simulink model "roll_ap"  (R2017b)
settings: Solver=FixedStepDiscrete  StartTime=0.0  StopTime=25  FixedStep=1/40  RelTol=1e-3
model workspace (MAT data in the model file):
  dispGain = Simulink.Parameter
  dispGain.Value = 1
  dispGain.DataType = 'auto'
  dispGain.Dimensions = [1 1]
  hdgGain = Simulink.Parameter
  hdgGain.Value = 0.015
  hdgGain.DataType = 'auto'
  hdgGain.Min = 0
  hdgGain.Dimensions = [1 1]
  intGain = Simulink.Parameter
  intGain.Value = 1
  intGain.DataType = 'auto'
  intGain.Dimensions = [1 1]
  rateGain = Simulink.Parameter
  rateGain.Value = 3
  rateGain.DataType = 'auto'
  rateGain.Dimensions = [1 1]
undefined symbols (not defined in the file or in its folder): cmdLim, dispLim, intLim, rateLim
libraries: simulink x1, simulink_need_slupdate x1
settings Model: RequirementInfo={} %GIDa_fe9045fd_0412_4b6e_8206_617cc20e6fde  ParameterArgumentNames=dispGain,intGain,rateGain,hdgGain  Creator=bpotter  LastModifiedBy=Hualong Yu
settings DataIOCC: ExternalInput=rollIn  SaveFormat=StructureWithTime  SignalLoggingSaveFormat=ModelDataLogs  SaveOutput=off  SignalLogging=off  SaveTime=off  OutputSaveName=Ail_Cmd
settings OptimizationCC: BlockReduction=off  DefaultParameterBehavior=Inlined  InlineInvariantSignals=on  ExpressionDepthLimit=2147483647  EfficientFloat2IntCast=on  EfficientMapNaN2IntZero=off  LifeSpan=inf  MaxStackSize=inf
settings DebuggingCC: SignalInfNanChecking=error  SignalRangeChecking=error  ReadBeforeWriteMsg=EnableAllAsError  WriteAfterWriteMsg=EnableAllAsError  WriteAfterReadMsg=EnableAllAsError  AlgebraicLoopMsg=error  ArtificialAlgebraicLoopMsg=error  SaveWithDisabledLinksMsg=error  SaveWithParameterizedLinksMsg=error  CheckExecutionContextPreStartOutputMsg=on  CheckExecutionContextRuntimeOutputMsg=on  BlockPriorityViolationMsg=error  MaxConsecutiveZCsMsg=warning  SolverPrmCheckMsg=error  InheritedTsInSrcMsg=error  SingleTaskRateTransMsg=error  TasksWithSamePriorityMsg=error  SigSpecEnsureSampleTimeMsg=error  CheckMatrixSingularityMsg=error  IntegerOverflowMsg=error  ParameterUnderflowMsg=error  ParameterPrecisionLossMsg=error  ParameterTunabilityLossMsg=error  UnderSpecifiedDataTypeMsg=error  UnnecessaryDatatypeConvMsg=warning  VectorMatrixConversionMsg=error  SignalLabelMismatchMsg=error  UnconnectedInputMsg=error  UnconnectedOutputMsg=error  UnconnectedLineMsg=error  SFcnCompatibilityMsg=error  UniqueDataStoreMsg=error  BusObjectLabelMismatch=error  RootOutportRequireBusObject=error  AssertControl=DisableAll  ModelReferenceIOMsg=error  ModelReferenceIOMismatchMessage=error  UnknownTsInhSupMsg=error  ModelReferenceDataLoggingMessage=error  ModelReferenceExtraNoncontSigs=none  StateNameClashWarn=warning  StrictBusMsg=ErrorOnBusTreatedAsVector  NonBusSignalsTreatedAsBus=error  SFUnexpectedBacktrackingDiag=warning  SFNoUnconditionalDefaultTransitionDiag=warning  SFExecutionAtInitializationDiag=none  IntegerSaturationMsg=error
settings HardwareCC: ProdBitPerPointer=32  ProdBitPerSizeT=32  ProdBitPerPtrDiffT=32  ProdLargestAtomicFloat=None  ProdEndianess=BigEndian  ProdWordSize=32  ProdHWDeviceType=32-bit Embedded Processor  TargetHWDeviceType=32-bit Generic
settings ModelReferenceCC: PropagateSignalLabelsOutOfModel=off
settings SFSimCC: MATLABDynamicMemAlloc=off
settings RTWCC: SystemTargetFile=ert.tlc  GenCodeOnly=on  GenerateMakefile=off  TemplateMakefile=ert_default_tmf  GenerateReport=on  RTWVerbose=off  IncludeHyperlinkInReport=on  LaunchReport=on  GenerateTraceInfo=on  GenerateTraceReport=on  GenerateTraceReportSl=on  GenerateTraceReportSf=on  GenerateTraceReportEml=on
settings CodeAppCC: ForceParamTrailComments=on  IgnoreCustomStorageClasses=off  MaxIdLength=63  MangleLength=4  CustomSymbolStrType=$N$R$M  StateflowObjectComments=on  InternalIdentifier=Classic  ReqsInCode=on
settings ERTTargetCC: UtilityFuncGeneration=Shared location  MultiwordLength=2048  IncludeMdlTerminateFcn=off  GeneratePreprocessorConditionals=Disable all  SuppressErrorStatus=on  SupportAbsoluteTime=off  MultiInstanceERTCode=on  CodeInterfacePackaging=Reusable function  SupportNonFinite=off  SupportComplex=off  ParenthesesLevel=Maximum  MultiInstanceErrorCode=None  ERTCustomFileTemplate=example_file_process.tlc  PreserveExpressionOrder=on  PreserveIfCondition=on  ConvertIfToSwitch=off  SuppressUnreachableDefaultCases=off
settings ConfigComp: CovSaveName=covdata_rollAP  CovMetricSettings=dcmtrwe  CovHTMLOptions=-aTS=1 -bRG=1 -bTC=1 -hTR=1 -nFC=0 -scm=1 -bcm=1  CovSaveCumulativeToWorkspaceVar=on  CovSaveSingleToWorkspaceVar=on  CovCumulativeVarName=covCumulativeData_rollAP  CovCumulativeReport=on  CovReportOnPause=off  CovExternalEMLEnable=off

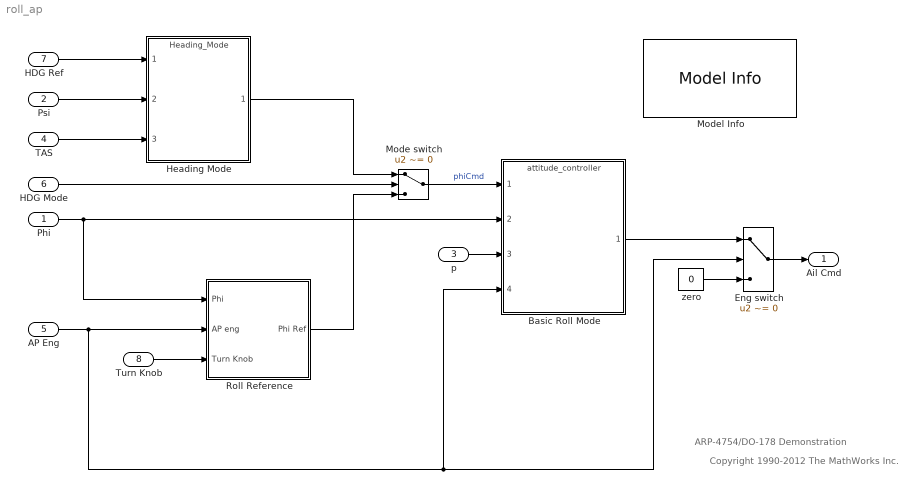
== system roll_ap ==
  note: Copyright 1990-2012 The MathWorks Inc.
  note: ARP-4754/DO-178 Demonstration
  Phi : Inport  RequirementInfo={} %GIDa_040c2d73_6311_42f9_964f_56f1fff3d8d8  OutDataTypeStr=double  PortDimensions=1  SampleTime=1/40  Interpolate=off
  Psi : Inport  RequirementInfo={} %GIDa_aa699f91_96f0_401b_acdb_f9b4b0743533  Port=2  OutDataTypeStr=double  PortDimensions=1  SampleTime=1/40  Interpolate=off
  p : Inport  RequirementInfo={} %GIDa_91b6e343_cedd_4c09_9e82_9cc09e4312a7  Port=3  OutDataTypeStr=double  PortDimensions=1  SampleTime=1/40  Interpolate=off
  TAS : Inport  RequirementInfo={} %GIDa_9daa2c3d_09c1_4ac6_a206_1425f5f778cd  Port=4  OutDataTypeStr=double  PortDimensions=1  SampleTime=1/40  Interpolate=off
  AP Eng : Inport  RequirementInfo={} %GIDa_dbf8c750_871c_42fc_8ea1_57838e97fa97  Port=5  OutDataTypeStr=boolean  PortDimensions=1  SampleTime=1/40  Interpolate=off
  HDG Mode : Inport  RequirementInfo={} %GIDa_3d1fd2be_b046_42ef_8f3c_1955bceadbb7  Port=6  OutDataTypeStr=boolean  PortDimensions=1  SampleTime=1/40  Interpolate=off
  HDG Ref : Inport  RequirementInfo={} %GIDa_96162cda_cb1a_490e_8dac_f861526aad50  Port=7  OutDataTypeStr=double  PortDimensions=1  SampleTime=1/40  Interpolate=off
  Turn Knob : Inport  RequirementInfo={} %GIDa_fa976ccd_1ea9_4823_b673_fef2768ad601  Port=8  OutDataTypeStr=double  PortDimensions=1  SampleTime=1/40  Interpolate=off
  Basic Roll Mode : ModelReference  RequirementInfo={} %GIDa_94fed7b0_f432_43f5_a2d9_2abccf075f5b  ModelNameDialog=attitude_controller  ParameterArgumentNames=cmdLim,dispGain,dispLim,intGain,intLim,rateGain,rateLim  ParameterArgumentValues=15,dispGain,30,intGain,5,rateGain,6  UsingDefaultArgumentValue=0,0,0,0,0,0,0  SimulationMode=Normal  ModelReferenceVersion=1.44
  Eng switch : Switch  RequirementInfo={} %GIDa_1f89e2a1_f10b_411b_80f1_4c7070559f04  Criteria=u2 ~= 0
  Heading Mode : ModelReference  RequirementInfo={} %GIDa_e0954c89_e814_46d2_8f67_6d4b1cdfab81  ModelNameDialog=Heading_Mode  ParameterArgumentNames=hdgGain  ParameterArgumentValues=hdgGain  UsingDefaultArgumentValue=0  SimulationMode=Normal  ModelReferenceVersion=1.133
  Mode switch : Switch  RequirementInfo={} %GIDa_89518de0_411a_4ee8_869d_c7ed5e5087e3  Criteria=u2 ~= 0
  Model Info : simulink/Model-Wide Utilities/Model Info  RequirementInfo={} %GIDa_ca11a4b2_f22f_461f_8532_eb2c7aa53101  Frame=on  DisplayStringWithTags=|  HorizontalTextAlignment=Left  LeftAlignmentValue=0.02
      | Roll Autopilot
      | Author: %<LastModifiedBy>
      | Model Version: %<ModelVersion>
      | Date: %<LastModificationDate>
  Roll Reference : Subsystem  TreatAsAtomicUnit=on
      settings: RTWSystemCode=Inline
  zero : Constant  RequirementInfo={} %GIDa_8c99e557_6257_4659_beae_770a67a6ac3a  Value=0  OutDataTypeStr=double
  Ail Cmd : Outport  RequirementInfo={} %GIDa_02b61f6d_71d4_4b0d_89ac_bfbca808eb5f  OutDataTypeStr=double  PortDimensions=1  SampleTime=1/40
  wires:
  HDG Ref/1 -> Heading Mode/1
  Phi/1 -> Roll Reference/1(Phi), Basic Roll Mode/2
  p/1 -> Basic Roll Mode/3
  Psi/1 -> Heading Mode/2
  TAS/1 -> Heading Mode/3
  Mode switch/1 -> Basic Roll Mode/1  "phiCmd"
  HDG Mode/1 -> Mode switch/2
  Heading Mode/1 -> Mode switch/1
  AP Eng/1 -> Eng switch/2, Basic Roll Mode/4, Roll Reference/2(AP eng)
  Basic Roll Mode/1 -> Eng switch/1
  Eng switch/1 -> Ail Cmd/1
  zero/1 -> Eng switch/3
  Roll Reference/1(Phi Ref) -> Mode switch/3
  Turn Knob/1 -> Roll Reference/3(Turn Knob)

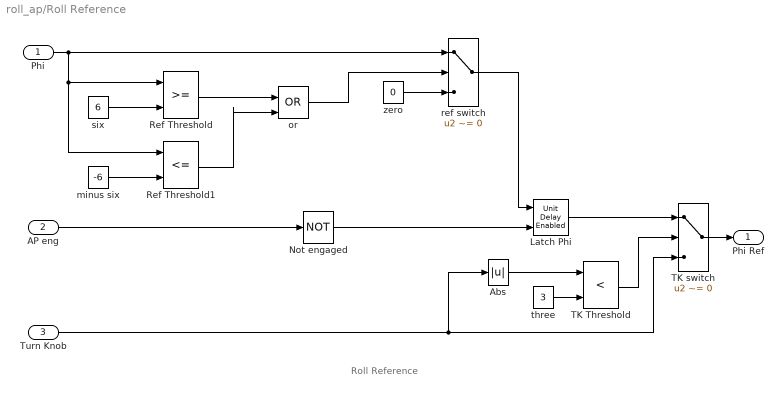
== system roll_ap/Roll Reference ==
  note: Roll Reference
  Phi : Inport
  AP eng : Inport  Port=2
  Turn Knob : Inport  Port=3
  Abs : Abs
  Latch Phi : simulink_need_slupdate/Unit Delay Enabled  RequirementInfo={} %GIDa_8c2a6474_62f7_4673_9b80_815aaee792d7  vinit=0.0  tsamp=1/40
      settings: SourceProductName=Simulink  SourceProductBaseCode=SL
  Not engaged : Logic  RequirementInfo={} %GIDa_e52c6893_d81b_4f15_89c3_12b6a83c27b2  Operator=NOT  IconShape=distinctive  AllPortsSameDT=off  OutDataTypeStr=boolean
  Ref Threshold : RelationalOperator  RequirementInfo={} %GIDa_be19764a_4253_499a_816c_5a218f85ba52  OutDataTypeStr=boolean  RndMeth=Nearest  InputSameDT=on
  Ref Threshold1 : RelationalOperator  RequirementInfo={} %GIDa_66db49a9_aa40_43ab_9d6f_efe68ac443ed  Operator=<=  OutDataTypeStr=boolean  RndMeth=Nearest  InputSameDT=on
  TK Threshold : RelationalOperator  RequirementInfo={} %GIDa_9859b478_272f_4974_a36c_6c4f8c030643  Operator=<  OutDataTypeStr=boolean  RndMeth=Nearest  InputSameDT=on
  TK switch : Switch  RequirementInfo={} %GIDa_804165d0_89eb_4919_a8d1_f2310004f7d9  Criteria=u2 ~= 0
  minus six : Constant  RequirementInfo={} %GIDa_3d290e71_7846_48ec_bba2_120ec195a4d2  Value=-6
  or : Logic  Operator=OR  IconShape=distinctive  OutDataTypeStr=boolean
  ref switch : Switch  RequirementInfo={} %GIDa_a4746381_6ebe_4e3d_83b9_b49d14a3af5e  Criteria=u2 ~= 0
  six : Constant  RequirementInfo={} %GIDa_0870d8d6_d29f_4cb4_9c0c_9079ccdb7173  Value=6
  three : Constant  RequirementInfo={} %GIDa_6228e2c4_8022_4eaf_90d6_7c47f19fb0a2  Value=3  OutDataTypeStr=double
  zero : Constant  RequirementInfo={} %GIDa_e4775650_e5c7_4c74_aef4_71c144af3cbc  Value=0
  Phi Ref : Outport
  wires:
  Not engaged/1 -> Latch Phi/2
  ref switch/1 -> Latch Phi/1
  Latch Phi/1 -> TK switch/1
  TK Threshold/1 -> TK switch/2
  Turn Knob/1 -> TK switch/3, Abs/1
  three/1 -> TK Threshold/2
  Abs/1 -> TK Threshold/1
  Phi/1 -> ref switch/1, Ref Threshold/1, Ref Threshold1/1
  AP eng/1 -> Not engaged/1
  TK switch/1 -> Phi Ref/1
  six/1 -> Ref Threshold/2
  zero/1 -> ref switch/3
  or/1 -> ref switch/2
  Ref Threshold/1 -> or/1
  Ref Threshold1/1 -> or/2
  minus six/1 -> Ref Threshold1/2
